simulink model "simrotor1"  (Simulink 3.00)
settings: Solver=ode23tb  SolverMode=SingleTasking  StartTime=0.0  StopTime=10.0  RelTol=1e-1  AbsTol=1e-1
undefined symbols (not defined in the file or in its folder): ar, br, cr, dr, full
libraries: simulink3 x1

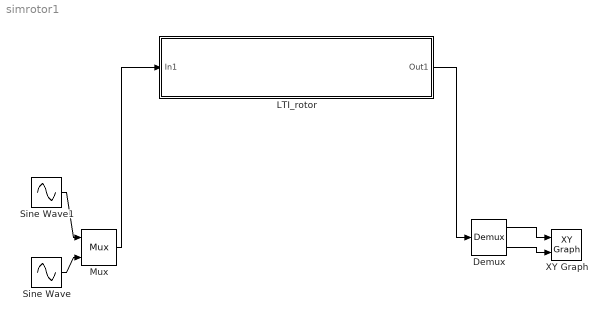
== system simrotor1 ==
  Demux : Demux  Outputs=2
  LTI_rotor : Subsystem  Description=Rotor Linear Model  mask{ModelName=simple2s, W=2500}
      mask prompts: ModelName "Model Template"; W "Speed of Rotation [RPM]"
      mask init:
      | Rot=rotfe(ModelName); [ar,br,cr,dr]=rot2ss(Rot,W*2*pi/60);
      mask Display: disp(ModelName)
  Mux : Mux  Inputs=2
      settings: DisplayOption=none
  Sine Wave : Sin  Amplitude=1000  Frequency=1  Phase=0  SampleTime=0
  Sine Wave1 : Sin  Amplitude=1000  Frequency=1  Phase=pi/2  SampleTime=0
  XY Graph : simulink3/Sinks/XY Graph  xmin=-1  xmax=1  ymin=-1  ymax=1  st=-1
  wires:
  LTI_rotor/1(Out1) -> Demux/1
  Demux/1 -> XY Graph/1
  Demux/2 -> XY Graph/2
  Mux/1 -> LTI_rotor/1(In1)
  Sine Wave/1 -> Mux/2
  Sine Wave1/1 -> Mux/1

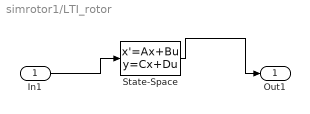
== system simrotor1/LTI_rotor ==
  In1 : Inport  Port=1  PortWidth=-1  SampleTime=-1  DataType=auto
      settings: SignalType=auto
  State-Space : StateSpace  A=full(ar)  B=full(br)  C=full(cr)  D=full(dr)  X0=0
  Out1 : Outport  Port=1
  wires:
  In1/1 -> State-Space/1
  State-Space/1 -> Out1/1
